simulink model "X8"  (R2020b)
settings: Solver=FixedStepAuto  StartTime=0.0  StopTime=Inf  FixedStep=1e-3  MinStep=0.0001  RelTol=1e-3  EnableMultiTasking=on
model workspace (MAT data in the model file):
  FaultMode = Simulink.Parameter
  FaultMode.Value = 0
  FaultMode.Description = 'Fault mode parameter object'
  FaultMode.DataType = 'auto'
  FaultMode.Dimensions = [1 1]
values from neighbouring files (symbols this model uses):
  A = [ ... (first row only)    [calc_sys_long.m]
  C_L_delta_eInterpolation = Create_interpolation(C_L_delta_e_data,'C_L_delta_e_data')    [coeff_ctrl.m]
  F = K * (-(C_D_0 + C_D_alpha * alpha) * cos(alpha)      + (C_L_O + C_L_alpha * alpha)*sin(alpha)) - f_x    [calc_alpha.m]
  h0 = 1000    [init.m]
  input_source = 4    [runX8.m]
  input_source0 = 1    [runX8.m]
  input_step_time = 0    [runX8.m]
  J = @(v_a, omega) 2 * pi * v_a / (omega*obj.prop_diam)    [kalmanFilters.m]    (also in motor.m = 2*pi*Va/omega/prop_diam; motor_fault.m = c2 / omega)
  lat0 = 37.6205    [init.m]
  lon0 = -122.3815    [init.m]
  P = filter.P(i,i,k_0:k_1)    [filterTest.m]    (also in kalmanFilters.m = filter.P)
  p = rate(1) + wind(4)    [forces.m]    (also in forces_trim.m)
  q = rate(2) + wind(5)    [forces.m]    (also in forces_trim.m)
  r = rate(3) + wind(6)    [forces.m]    (also in forces_trim.m)
  T_elevon2ailelev = [1 1 ... (first row only)    [init.m]
  Ts = 0.01    [init.m]
  U_trim = [op.Inputs(1).u;op.Inputs(2).u;op.Inputs(3).u;op.Inputs(4).u]    [X8Trim.m]
  x0 = X_trim    [X8Trim.m]    (also in init.m = [eta_0', ny_0' zeros(1,6)]'; runX8.m = [      0                 0                    -h_ini        ; trimX8.m = [      37.5                 0                    -h_ini     )
undefined symbols (not defined in the file or in its folder): Friction, ia, ib, interp_C_D_alpha, interp_C_D_delta_e, interp_C_D_q, interp_C_L_alpha, interp_C_l_beta, interp_C_l_delta_a, interp_C_L_delta_e, interp_C_l_delta_r, interp_C_l_p, interp_C_L_q, interp_C_l_r, interp_C_m_alpha, interp_C_m_delta_e, interp_C_m_q, interp_C_n_beta, interp_C_n_delta_a, interp_C_n_p, interp_C_n_r, interp_C_Y_beta, interp_C_Y_delta_a, interp_C_Y_delta_r, interp_C_Y_p, interp_C_Y_r, Ion, JSBSim, Light, Lithium, Lls, MIL, Prop_param, Rascal110, Receive, Rs, Send, Standard_Devices, thetam, UDP_Protocol, wm, x0_stationary
libraries: simulink_extras x15, simulink x8, aerolibwind2 x4, sldrtlib x3, aerolibfltsims x3, aerolibactuator x3, sharedtransform x3, electricdrivelib x2, dspnetwork x1, aerolibnav x1, sharedutil x1, powerlib_meascontrol x1
(part 1 of 2)
settings Model: SimulationMode=accelerator  PacingRate=10  ParameterArgumentNames=FaultMode  OrderedModelArguments=off  Creator=krisgry  LastModifiedBy=ole
settings SolverCC: ZeroCrossAlgorithm=Adaptive  AutoInsertRateTranBlk=on
settings DataIOCC: SaveOutput=off  DSMLogging=off  SaveTime=off  ReturnWorkspaceOutputs=off  LoggingFileName=simulationData.mat
settings OptimizationCC: EfficientMapNaN2IntZero=off  AccelVerboseBuild=on
settings DebuggingCC: ReadBeforeWriteMsg=DisableAll  WriteAfterWriteMsg=DisableAll  WriteAfterReadMsg=DisableAll  SolverPrmCheckMsg=warning  MultiTaskCondExecSysMsg=warning  SFUnexpectedBacktrackingDiag=warning  SFNoUnconditionalDefaultTransitionDiag=warning  SFExecutionAtInitializationDiag=none  ArithmeticOperatorsInVariantConditions=warning
settings HardwareCC: ProdBitPerLong=64  ProdHWDeviceType=Intel->x86-64 (Mac OS X)  TargetBitPerLong=64  TargetBitPerPointer=64  TargetBitPerSizeT=64  TargetBitPerPtrDiffT=64  TargetLongLongMode=on  TargetIntDivRoundTo=Zero  TargetEndianess=LittleEndian  TargetWordSize=64  TargetHWDeviceType=MATLAB Host  ProdEqTarget=off
settings ModelReferenceCC: PropagateSignalLabelsOutOfModel=off
settings SFSimCC: SimUseLocalCustomCode=off  CustomCodeUndefinedFunction=UseInterfaceOnly
settings CodeAppCC: MaxIdLength=128
settings GRTTargetCC: TargetLangStandard=C89/C90 (ANSI)  CombineOutputUpdateFcns=off  GRTInterface=on
settings ConfigComp: CovMetricSettings=dw  CovSaveCumulativeToWorkspaceVar=on  CovSaveSingleToWorkspaceVar=on  CovExternalEMLEnable=off  CovSFcnEnable=off

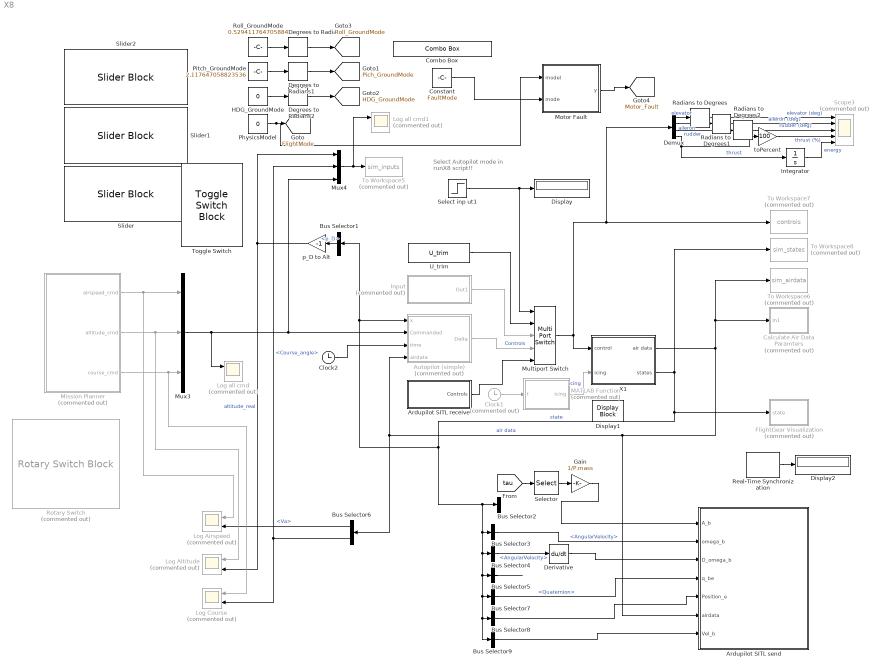
== system X8 ==
  note: Select Autopilot
      | mode in runX8 script!!
  Ardupilot SITL receive : Subsystem
  Ardupilot SITL send : Subsystem
  Autopilot (simple) : Subsystem  Commented=on
  Bus Selector1 : BusSelector  OutputSignals=Position.p_D
  Bus Selector2 : BusSelector  OutputSignals=Acceleration
  Bus Selector3 : BusSelector  OutputSignals=AngularVelocity
  Bus Selector4 : BusSelector  OutputSignals=AngularVelocity
  Bus Selector5 : BusSelector  OutputSignals=Velocity.u,Velocity.v,Velocity.w  OutputAsBus=on
  Bus Selector6 : BusSelector  OutputSignals=Va,Course_angle
  Bus Selector7 : BusSelector  OutputSignals=Quaternion
  Bus Selector8 : BusSelector  OutputSignals=Position.p_N,Position.p_E,Position.p_D  OutputAsBus=on
  Bus Selector9 : BusSelector  OutputSignals=Velocity.u,Velocity.v,Velocity.w  OutputAsBus=on
  Calculate Air Data Paramters : Subsystem  Commented=on
  Clock1 : Clock  Commented=on
  Clock2 : Clock
  Combo Box : ComboBox  LabelPosition=Hide  SelectedLabel=Mode 0
      settings: Values={{'Mode 0', 'Mode 1', 'Mode 2', 'Mode 3'}, [0 1 2 3]}
  Constant : Constant  Value=FaultMode
  Degrees to Radians : simulink_extras/Transformations/Degrees to Radians
  Degrees to Radians1 : simulink_extras/Transformations/Degrees to Radians
  Degrees to Radians2 : simulink_extras/Transformations/Degrees to Radians
  Demux : Demux
  Derivative : Derivative
  Display : Display
  Display1 : DisplayBlock
  Display2 : Display
  "FlightGear Visualization " : Subsystem  Commented=on
  Gain : Gain  Gain=1/P.mass
  HDG_GroundMode : Constant  Value=0  SampleTime=-1
  Input : Subsystem  Commented=on
  Integrator : Integrator
  Log Airspeed : Scope  Commented=on  NumInputPorts=2
  Log Altitude : Scope  Commented=on  NumInputPorts=2
  Log Course : Scope  Commented=on  NumInputPorts=2
  Log all cmd : Scope  Commented=on  NumInputPorts=2
  Log all cmd1 : Scope  Commented=on  NumInputPorts=2
  MATLAB Function : MATLAB Function  Commented=on  TreatAsAtomicUnit=on
  Mission Planner : Subsystem  Commented=on
  Motor Fault : MATLAB Function  TreatAsAtomicUnit=on
  Multiport Switch : MultiPortSwitch  Inputs=4
  Mux3 : Mux  Inputs=3
  Mux4 : Mux  Inputs=3
  PhysicsModel : Constant  Value=0  SampleTime=[0,1]
  Pitch_GroundMode : Constant  Value=2.117647058823536  SampleTime=-1
  Radians to Degrees : simulink_extras/Transformations/Radians to Degrees
  Radians to Degrees1 : simulink_extras/Transformations/Radians to Degrees
  Radians to Degrees2 : simulink_extras/Transformations/Radians to Degrees
  Real-Time Synchronization : sldrtlib/Real-Time Synchronization  SampleTime=0.1  MaxMissedTicks=inf  ShowMissedTicks=on  YieldWhenWaiting=off
  Roll_GroundMode : Constant  Value=0.529411764705884  SampleTime=-1
  Rotary Switch : RotarySwitchBlock  Commented=on
      settings: Values={{'Off', 'K_E', 'R_E', 'icing', 'off', 'I_0', 'c_v'}, [0 1 2 3 4 5 6]}
  Scope3 : Scope  Commented=on  NumInputPorts=5
  Select inp ut1 : Step  Time=input_step_time  Before=input_source0  After=input_source  SampleTime=0
  Selector : Selector  InputPortWidth=6  IndexOptions=Index vector (dialog)  Indices=[1 2 3]  OutputSizes=1
  Slider : SliderBlock  ScaleMax=360
  Slider1 : SliderBlock  ScaleMin=-180  ScaleMax=180
  Slider2 : SliderBlock  ScaleMin=-90  ScaleMax=90
  To Workspace5 : ToWorkspace  Commented=on  VariableName=sim_inputs  SaveFormat=Timeseries  SampleTime=-1
  To Workspace6 : ToWorkspace  Commented=on  VariableName=sim_airdata  SaveFormat=Timeseries  SampleTime=-1
  To Workspace7 : ToWorkspace  Commented=on  VariableName=controls  SaveFormat=Timeseries  SampleTime=-1
  To Workspace8 : ToWorkspace  Commented=on  VariableName=sim_states  SaveFormat=Timeseries  SampleTime=-1
  Toggle Switch : ToggleSwitchBlock
      settings: Values={{'Ground', 'Fly'}, [0 1]}
  U_trim : Constant  Value=U_trim  SampleTime=-1
  X1 : Subsystem
  p_D to Alt : Gain  Gain=-1
  toPercent : Gain  Gain=100
  tag scope: FlightMode=global, HDG_GroundMode=global, Motor_Fault=global, Pich_GroundMode=global, Roll_GroundMode=global
  wires:
  X1/1(air data) -> Autopilot (simple)/4(airdata), Bus Selector6/1, Ardupilot SITL send/6(airdata), Calculate Air Data Paramters/1(In1), To Workspace6/1  "air data"
  Multiport Switch/1 -> X1/1(control), To Workspace7/1, Demux/1
  U_trim/1 -> Multiport Switch/2
  Input/1(Out1) -> Multiport Switch/3
  X1/2(states) -> Bus Selector2/1, Bus Selector9/1, Bus Selector8/1, Bus Selector7/1, Bus Selector5/1, Bus Selector4/1, Bus Selector3/1, Bus Selector1/1, Autopilot (simple)/1(x), "FlightGear Visualization "/1(state), To Workspace8/1  "state"
  Select inp ut1/1 -> Multiport Switch/1, Display/1
  Mux3/1 -> Log all cmd/1, Mux4/3, Autopilot (simple)/2(Commanded)
  Autopilot (simple)/1(Delta) -> Multiport Switch/4  "Controls"
  Bus Selector6/2 -> Log Course/2, Mux4/2  "<Course_angle>"
  Bus Selector1/1 -> p_D to Alt/1  "<p_D>"
  p_D to Alt/1 -> Log Altitude/2, Mux4/1  "altitude_real"
  Mux4/1 -> Log all cmd1/1, To Workspace5/1
  Bus Selector6/1 -> Log Airspeed/2  "<Va>"
  Mission Planner/1(airspeed_cmd) -> Mux3/1, Log Airspeed/1
  Mission Planner/3(course_cmd) -> Log Course/1, Mux3/3
  Mission Planner/2(altitude_cmd) -> Log Altitude/1, Mux3/2
  Demux/1 -> Radians to Degrees/1  "elevator"
  Demux/2 -> Radians to Degrees1/1  "aileron"
  Demux/3 -> Radians to Degrees2/1  "rudder"
  Demux/4 -> Integrator/1, toPercent/1  "thrust"
  Integrator/1 -> Scope3/5  "energy"
  Bus Selector3/1 -> Ardupilot SITL send/2(omega_b)  "<AngularVelocity>"
  Bus Selector4/1 -> Derivative/1  "<AngularVelocity>"
  Bus Selector7/1 -> Ardupilot SITL send/4("q_be ")  "<Quaternion>"
  Bus Selector8/1 -> Ardupilot SITL send/5(Position_e)
  Derivative/1 -> Ardupilot SITL send/3(D_omega_b)
  Ardupilot SITL receive/1(Controls) -> Multiport Switch/5
  MATLAB Function/1(icing) -> X1/2(icing)  "icing"
  Clock1/1 -> MATLAB Function/1(t)
  Radians to Degrees/1 -> Scope3/1  "elevator (deg)"
  Radians to Degrees1/1 -> Scope3/2  "aileron (deg)"
  Radians to Degrees2/1 -> Scope3/3  "rudder (deg)"
  toPercent/1 -> Scope3/4  "thrust (%)"
  PhysicsModel/1 -> Motor Fault/1(model), [FlightMode]
  Pitch_GroundMode/1 -> Degrees to Radians1/1
  HDG_GroundMode/1 -> Degrees to Radians2/1
  Roll_GroundMode/1 -> Degrees to Radians/1
  Degrees to Radians/1 -> [Roll_GroundMode]
  Degrees to Radians1/1 -> [Pich_GroundMode]
  Degrees to Radians2/1 -> [HDG_GroundMode]
  Clock2/1 -> Autopilot (simple)/3(time)
  Gain/1 -> Ardupilot SITL send/1(A_b)
  Real-Time Synchronization/1 -> Display2/1
  Bus Selector5/1 -> ?
  Bus Selector9/1 -> Ardupilot SITL send/7(Vel_b)
  [tau] -> Selector/1
  Selector/1 -> Gain/1
  Motor Fault/1(y) -> [Motor_Fault]
  Constant/1 -> Motor Fault/2(mode)

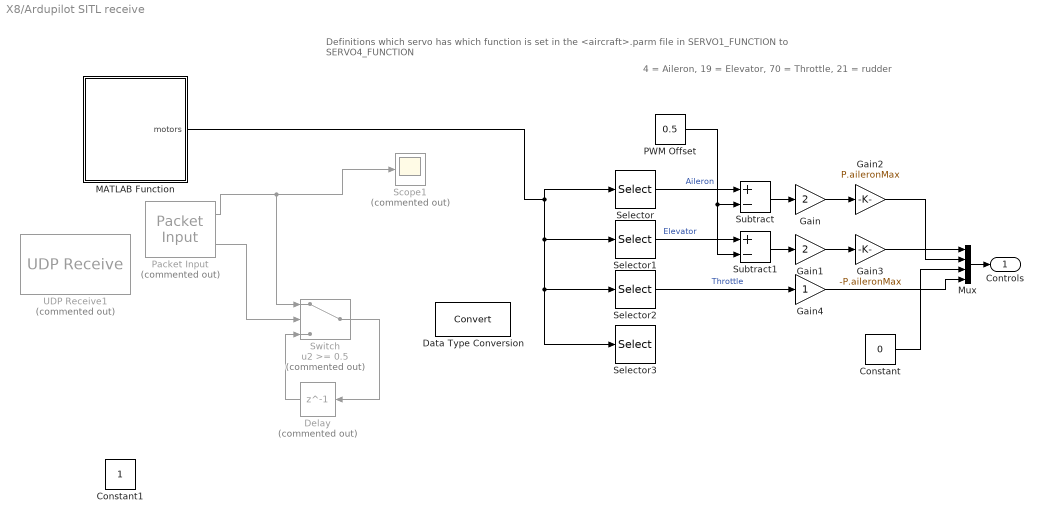
== system X8/Ardupilot SITL receive ==
  note: Definitions which servo has which function is set in the <aircraft>.parm file in SERVO1_FUNCTION to SERVO4_FUNCTION
  note: 4 = Aileron, 19 = Elevator, 70 = Throttle, 21 = rudder
  Constant : Constant  Value=0
  Constant1 : Constant
  Data Type Conversion : DataTypeConversion
  Delay : Delay  Commented=on  DelayLength=1  InitialCondition=0
  Gain : Gain  Gain=2
  Gain1 : Gain  Gain=2
  Gain2 : Gain  Gain=P.aileronMax
  Gain3 : Gain  Gain=-P.aileronMax
  Gain4 : Gain
  MATLAB Function : MATLAB Function  TreatAsAtomicUnit=on  SystemSampleTime=0.02
  Mux : Mux
  PWM Offset : Constant  Value=0.5
  Packet Input : sldrtlib/Packet Input  Commented=on  SampleTime=0.002  MaxMissedTicks=inf  ShowMissedTicks=off  YieldWhenWaiting=on  DrvName=Standard_Devices/UDP_Protocol  DrvAddress=9002  DrvOptions=[0 16385 0 0 0 0 0 0 0 0 0 0 0 0 0 0 0 0 0 0 0 0 0 0 0 0 0 0 0 0 0 0 0 0 0 0 0 0 0 0 0 0 0 0 0 0 0 0 0 0 0 0 0 0 0 0 0 0 0 0 0 0 0 0 0 0 0 0 0 0 0 0 0 0 0 0 0 0 0 0 0 0 0 0 0 0 0 0 0 0 0 0 0 0 0 0 0 0 0 0 0 0 0 0 0 0 0 0 0 0 0 0 0 0 0 0 0 0 0 0 0 0 0 0 0 0 0 0 0 0 0 0 0 0 0 0 0 0 0 0 0 0 0 0 0 0 0 0 0 0 0 0 0 0 0 0 0 0 0 0 0 0 0 0 0 0 0 0 0 0 0 0 0 0 0 0 0 0 0 0 0 0 0 0 0 0 0 0 0 0 0 0 0 0 0 0 0 0 0 0 0 0 0 0 0 0 0 0 0 0 0 0 0 0 0 0 0 0 0 0 0 0 0 0 0 0 0 0 0 0 0 0 0 0 0 0 0 0 0 0 0 0 0 0 0 0 0 0 0 0 0 0 0 0 0 0]  PacketSize=64  DataTypes='16*single'  ShowReady=on  ShowError=off  PacketID=1  ByteOrder=1  ShowTimestamp=off
      settings: AttributesFormatString=UDP Protocol [9002]
  Scope1 : Scope  Commented=on
  Selector : Selector  InputPortWidth=16  IndexOptions=Index vector (dialog)  Indices=1  OutputSizes=1
  Selector1 : Selector  InputPortWidth=16  IndexOptions=Index vector (dialog)  Indices=2  OutputSizes=1
  Selector2 : Selector  InputPortWidth=16  IndexOptions=Index vector (dialog)  Indices=3  OutputSizes=1
  Selector3 : Selector  InputPortWidth=16  IndexOptions=Index vector (dialog)  Indices=4  OutputSizes=1
  Subtract : Sum  Inputs=+-
  Subtract1 : Sum  Inputs=+-
  Switch : Switch  Commented=on  Threshold=0.5
  UDP Receive1 : dspnetwork/UDP Receive  Commented=on  localURL='0.0.0.0'  localPort=9002  remoteURL='127.0.0.1'  remotePort=-1  recvBufferSize=256  dims=16  signalDatatype=single  isComplex=off  isVarSize=off  showBlockingTime=on  blockingTime=0.02  sampletime=0.01  blockPlatform=HOST
  Controls : Outport  VectorParamsAs1DForOutWhenUnconnected=off
  wires:
  Selector2/1 -> Gain4/1  "Throttle"
  Mux/1 -> Controls/1
  Selector/1 -> Subtract/1  "Aileron"
  Selector1/1 -> Subtract1/1  "Elevator"
  PWM Offset/1 -> Subtract1/2, Subtract/2
  Subtract/1 -> Gain/1
  Subtract1/1 -> Gain1/1
  Gain1/1 -> Gain3/1
  Gain/1 -> Gain2/1
  Gain3/1 -> Mux/1
  Constant/1 -> Mux/3
  Gain2/1 -> Mux/2
  Gain4/1 -> Mux/4
  MATLAB Function/1(motors) -> Selector/1, Selector2/1, Selector3/1, Selector1/1
  Packet Input/1 -> Switch/1, Scope1/1
  Switch/1 -> Delay/1
  Packet Input/2 -> Switch/2
  Delay/1 -> Switch/3

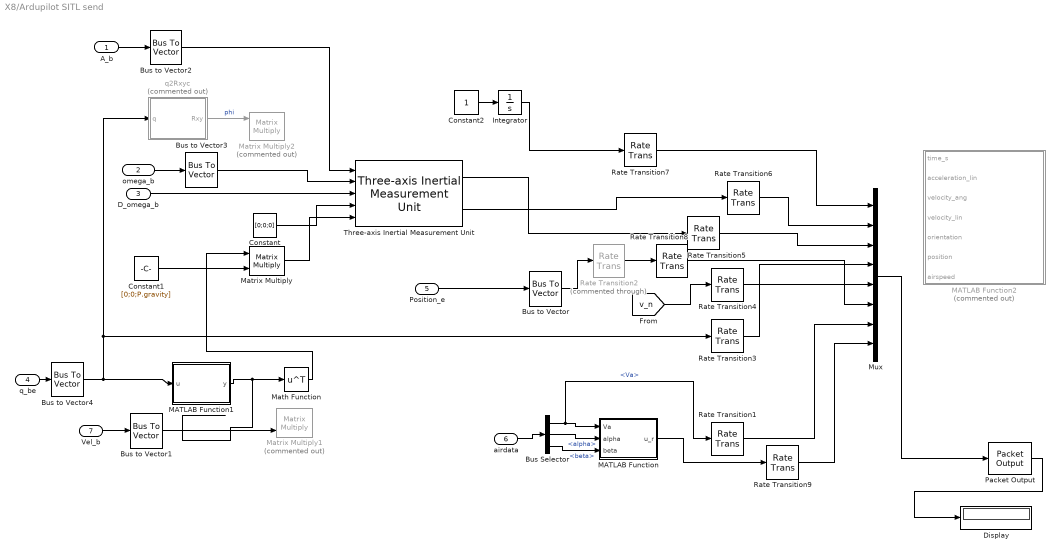
== system X8/Ardupilot SITL send ==
  A_b : Inport
  omega_b : Inport  Port=2
  D_omega_b : Inport  Port=3
  "q_be " : Inport  Port=4
  Position_e : Inport  Port=5
  airdata : Inport  Port=6
  Vel_b : Inport  Port=7
  Bus Selector : BusSelector  OutputSignals=Va,alpha,beta
  Bus to Vector{,1..4} (5 alike) : BusToVector
  Constant : Constant  Value=[0;0;0]
  Constant1 : Constant  Value=[0;0;P.gravity]
  Constant2 : Constant
  Display : Display
  Integrator : Integrator
  MATLAB Function : MATLAB Function  TreatAsAtomicUnit=on
  MATLAB Function1 : MATLAB Function  TreatAsAtomicUnit=on
  MATLAB Function2 : MATLAB Function  Commented=on  TreatAsAtomicUnit=on  SystemSampleTime=0.002
  Math Function : Math  Operator=transpose  SignedPower=on  SaturateOnIntegerOverflow=on
  Matrix Multiply : Product  Multiplication=Matrix(*)
  Matrix Multiply1 : Product  Commented=on  Multiplication=Matrix(*)
  Matrix Multiply2 : Product  Commented=on  Multiplication=Matrix(*)
  Mux : Mux  Inputs=8
  Packet Output : sldrtlib/Packet Output  SampleTime=0.002  MaxMissedTicks=inf  ShowMissedTicks=on  YieldWhenWaiting=off  DrvName=Standard_Devices/UDP_Protocol  DrvAddress=16384  DrvOptions=[0 9003 49 50 55 46 48 46 48 46 49 0 0 0 0 0 0 0 0 0 0 0 0 0 0 0 0 0 0 0 0 0 0 0 0 0 0 0 0 0 0 0 0 0 0 0 0 0 0 0 0 0 0 0 0 0 0 0 0 0 0 0 0 0 0 0 0 0 0 0 0 0 0 0 0 0 0 0 0 0 0 0 0 0 0 0 0 0 0 0 0 0 0 0 0 0 0 0 0 0 0 0 0 0 0 0 0 0 0 0 0 0 0 0 0 0 0 0 0 0 0 0 0 0 0 0 0 0 0 0 0 0 0 0 0 0 0 0 0 0 0 0 0 0 0 0 0 0 0 0 0 0 0 0 0 0 0 0 0 0 0 0 0 0 0 0 0 0 0 0 0 0 0 0 0 0 0 0 0 0 0 0 0 0 0 0 0 0 0 0 0 0 0 0 0 0 0 0 0 0 0 0 0 0 0 0 0 0 0 0 0 0 0 0 0 0 0 0 0 0 0 0 0 0 0 0 0 0 0 0 0 0 0 0 0 0 0 0 0 0 0 0 0 0 0 0 0 0 0 0 0 0 0 0 0 0]  PacketSize=176  DataTypes='22*double'  ShowReady=off  ShowError=off  PacketID=1  ByteOrder=1  InitialValue=[]  FinalValue=[]
      settings: AttributesFormatString=UDP Protocol [16384]
  Rate Transition{1,5..7} (4 alike) : RateTransition
  Rate Transition2 : RateTransition  Commented=through
  Rate Transition{3..4,8..9} (4 alike) : RateTransition  OutPortSampleTimeOpt=Inherit
  Three-axis Inertial Measurement Unit : aerolibnav/Three-axis Inertial Measurement Unit  units=Metric (MKS)  imu=[0 0 0]  i_Ts=0.001  dtype_a=off  w_a=190  z_a=0.707  a_sf_cc=[1 0 0; 0 1 0; 0 0 1]  a_bias=[0 0 0]  a_sat="[-inf  -inf  -inf  inf inf inf]"  dtype_g=off  w_g=190  z_g=0.707  g_sf_cc=[1 0 0; 0 1 0; 0 0 1]  g_bias=[0 0 0]  g_sens=[0 0 0]  g_sat="[-inf  -inf  -inf  inf inf inf]"  i_rand=off  i_seeds=[23093 23094 23095 23096 23097 23098]  i_pow=[0.001 0.001 0.001 0.0001 0.0001 0.0001]
  q2Rxyc : MATLAB Function  Commented=on  TreatAsAtomicUnit=on
  wires:
  Position_e/1 -> Bus to Vector/1
  airdata/1 -> Bus Selector/1
  Rate Transition2/1 -> Rate Transition8/1
  Bus Selector/1 -> Rate Transition1/1, MATLAB Function/1(Va)  "<Va>"
  A_b/1 -> Bus to Vector2/1
  D_omega_b/1 -> Three-axis Inertial Measurement Unit/3
  Constant/1 -> Three-axis Inertial Measurement Unit/4
  MATLAB Function1/1(y) -> Math Function/1
  Integrator/1 -> Rate Transition7/1
  Three-axis Inertial Measurement Unit/2 -> Rate Transition6/1
  Bus to Vector2/1 -> Three-axis Inertial Measurement Unit/1
  Constant1/1 -> Matrix Multiply/2
  Matrix Multiply/1 -> Three-axis Inertial Measurement Unit/5
  Bus to Vector/1 -> Rate Transition2/1
  Three-axis Inertial Measurement Unit/1 -> Rate Transition5/1
  Rate Transition7/1 -> Mux/1
  Rate Transition6/1 -> Mux/2
  Rate Transition5/1 -> Mux/3
  Rate Transition1/1 -> Mux/7
  Mux/1 -> Packet Output/1
  Packet Output/1 -> Display/1
  Bus Selector/2 -> MATLAB Function/2(alpha)  "<alpha>"
  Bus Selector/3 -> MATLAB Function/3(beta)  "<beta>"
  MATLAB Function/1(u_r) -> Rate Transition9/1
  Vel_b/1 -> Bus to Vector1/1
  ? -> Matrix Multiply1/1
  Bus to Vector1/1 -> Matrix Multiply1/2
  [v_n] -> Rate Transition4/1
  Constant2/1 -> Integrator/1
  Math Function/1 -> Matrix Multiply/1
  q2Rxyc/1(Rxy) -> Matrix Multiply2/1  "phi"
  omega_b/1 -> Bus to Vector3/1
  Bus to Vector3/1 -> Three-axis Inertial Measurement Unit/2
  "q_be "/1 -> Bus to Vector4/1
  Bus to Vector4/1 -> MATLAB Function1/1(u), q2Rxyc/1(q), Rate Transition3/1
  Rate Transition3/1 -> Mux/4
  Rate Transition8/1 -> Mux/6
  Rate Transition4/1 -> Mux/5
  Rate Transition9/1 -> Mux/8

== system X8/Autopilot (simple) ==
  x : Inport
  Commanded : Inport  Port=2
  time : Inport  Port=3
  airdata : Inport  Port=4
  Bus Selector : BusSelector  OutputSignals=Va,alpha,beta,wind_x,wind_y,wind_z,Course_angle
  Bus Selector1 : BusSelector  OutputSignals=Position.p_N,Position.p_E,Position.p_D,Velocity.u,Velocity.v,Velocity.w,Attitude.phi,Attitude.theta,Attitude.psi,AngularVelocity.p,AngularVelocity.q,AngularVelocity.r
  Delay : Delay  DelayLength=1  InitialCondition="[x0(1:3);  x0(8:10); zeros(3,1); x0(11:13); zeros(11,1)]"  SampleTime=Ts
  Interpreted MATLAB Function : MATLABFcn  MATLABFcn=autopilot  OutputDimensions=4
  Memory : Memory  Commented=on  InitialCondition="[x0(1:3);  x0(8:10); zeros(3,1); x0(11:13); zeros(11,1)]"
  Mux : Mux
  Mux1 : Mux  Inputs=7
  Mux2 : Mux  Inputs=12
  To Workspace1 : ToWorkspace  VariableName=commanded  SaveFormat=Structure With Time  SampleTime=-1
  To Workspace2 : ToWorkspace  VariableName=delta  SaveFormat=Structure With Time  SampleTime=-1
  Delta : Outport  VectorParamsAs1DForOutWhenUnconnected=off
  wires:
  Commanded/1 -> To Workspace1/1, Mux/2
  Mux/1 -> Delay/1
  time/1 -> Mux/4
  airdata/1 -> Bus Selector/1
  Bus Selector/1 -> Mux1/1  "<Va>"
  Bus Selector/2 -> Mux1/2  "<alpha>"
  Bus Selector/3 -> Mux1/3  "<beta>"
  Bus Selector/4 -> Mux1/4  "<wind_x>"
  Bus Selector/5 -> Mux1/5  "<wind_y>"
  Bus Selector/6 -> Mux1/6  "<wind_z>"
  Mux1/1 -> Mux/3
  x/1 -> Bus Selector1/1
  Bus Selector1/1 -> Mux2/1  "<p_N>"
  Bus Selector1/2 -> Mux2/2  "<p_E>"
  Bus Selector1/4 -> Mux2/4  "<u>"
  Bus Selector1/3 -> Mux2/3  "<p_D>"
  Bus Selector1/5 -> Mux2/5  "<v>"
  Bus Selector1/6 -> Mux2/6  "<w>"
  Bus Selector1/7 -> Mux2/7  "<phi>"
  Bus Selector1/9 -> Mux2/9  "<psi>"
  Bus Selector1/8 -> Mux2/8  "<theta>"
  Bus Selector1/10 -> Mux2/10  "<p>"
  Bus Selector1/11 -> Mux2/11  "<q>"
  Bus Selector1/12 -> Mux2/12  "<r>"
  Mux2/1 -> Mux/1
  Interpreted MATLAB Function/1 -> To Workspace2/1, Delta/1
  Delay/1 -> Interpreted MATLAB Function/1
  Bus Selector/7 -> Mux1/7  "<Course_angle>"

== system X8/Calculate Air Data Paramters ==
  In1 : Inport
  Bus Selector : BusSelector  OutputSignals=alpha,beta,Va
  Radians to Degrees1 : simulink_extras/Transformations/Radians to Degrees
  Radians to Degrees4 : simulink_extras/Transformations/Radians to Degrees
  To Workspace : ToWorkspace  VariableName=alpha  SaveFormat=Structure With Time  SampleTime=-1
  To Workspace1 : ToWorkspace  VariableName=beta  SaveFormat=Structure With Time  SampleTime=-1
  To Workspace2 : ToWorkspace  VariableName=va  SaveFormat=Structure With Time  SampleTime=-1
  wires:
  Radians to Degrees1/1 -> To Workspace1/1  "beta_ref"
  Radians to Degrees4/1 -> To Workspace/1  "alpha_ref"
  In1/1 -> Bus Selector/1
  Bus Selector/2 -> Radians to Degrees1/1  "<beta>"
  Bus Selector/1 -> Radians to Degrees4/1  "<alpha>"
  Bus Selector/3 -> To Workspace2/1  "<Va>"

== system X8/FlightGear Visualization  ==
  state : Inport
  Bus Selector : BusSelector  OutputSignals=Attitude  OutputAsBus=on
  Bus Selector2 : BusSelector  OutputSignals=Position
  "FlatEarth to Lon/Lat/Alt " : Subsystem
  FlightGear Preconfigured 6DoF Animation : aerolibfltsims/FlightGear Preconfigured 6DoF Animation  xFlightGearVersion=v2018.1  DestinationIpAddress=127.0.0.1  DestinationPort=5600  SampleTime=0.02  packetVersion=24
  Generate Run Script : aerolibfltsims/Generate Run Script  Architecture=Linux  dataFlow=Send  GeometryModelName=Rascal110-JSBSim  AirportId=KSFO  RunwayId=10L  InitialAltitude=7224  InitialHeading=113  OffsetDistance=4.72  OffsetAzimuth=0  InstallScenery=off  DisableShaders=off  OriginAddress=127.0.0.1  DestinationPort=5600  OriginPort=5505  LocalAddress=127.0.0.1  OutputFileName=runfg.sh  FlightGearBaseDirectory=/home/adrian/.fgfs
  "Initial position (lon (°), lat (°), alt (m)) " : Constant  Value=[lon0, lat0, h0]  VectorParams1D=off
  Mux : Mux  Inputs=2
  wires:
  Mux/1 -> FlightGear Preconfigured 6DoF Animation/1
  Bus Selector2/1 -> "FlatEarth to Lon/Lat/Alt "/1("DeltaPosition [N (m), E(m), D(m)]")  "<Position>"
  state/1 -> Bus Selector2/1, Bus Selector/1
  "FlatEarth to Lon/Lat/Alt "/1(Out1) -> Mux/1
  Bus Selector/1 -> Mux/2  "<signal2>"
  "Initial position (lon (°), lat (°), alt (m)) "/1 -> "FlatEarth to Lon/Lat/Alt "/2("InitPosition [N (°), E(°), Alt (m)] ")

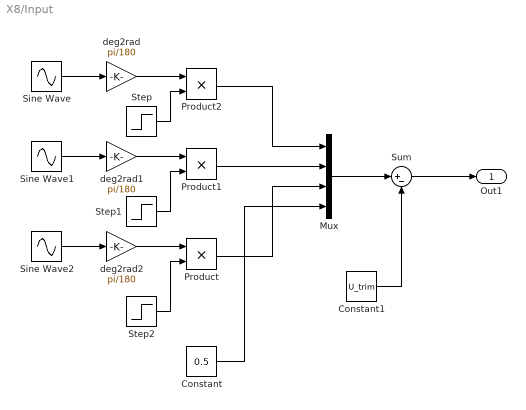
== system X8/Input ==
  Constant : Constant  Value=0.5
  Constant1 : Constant  Value=U_trim
  Mux : Mux
  Product : Product
  Product1 : Product
  Product2 : Product
  Sine Wave : Sin  Amplitude=1e-3  Frequency=0.1  SampleTime=0
  Sine Wave1 : Sin  Amplitude=1e-4  Frequency=0.01  Phase=pi/2  SampleTime=0
  Sine Wave2 : Sin  Amplitude=1e-3  Frequency=0.05  Phase=pi  SampleTime=0
  Step : Step  SampleTime=0
  Step1 : Step  Time=50  SampleTime=0
  Step2 : Step  Time=100  SampleTime=0
  Sum : Sum  Inputs=|+-
  deg2rad : Gain  Gain=pi/180
  deg2rad1 : Gain  Gain=pi/180
  deg2rad2 : Gain  Gain=pi/180
  Out1 : Outport  VectorParamsAs1DForOutWhenUnconnected=off
  wires:
  Sine Wave/1 -> deg2rad/1
  Sine Wave1/1 -> deg2rad1/1
  Sine Wave2/1 -> deg2rad2/1
  deg2rad2/1 -> Product/1
  deg2rad1/1 -> Product1/1
  deg2rad/1 -> Product2/1
  Step/1 -> Product2/2
  Step1/1 -> Product1/2
  Step2/1 -> Product/2
  Product2/1 -> Mux/1
  Product1/1 -> Mux/2
  Product/1 -> Mux/3
  Constant/1 -> Mux/4
  Mux/1 -> Sum/1
  Sum/1 -> Out1/1
  Constant1/1 -> Sum/2

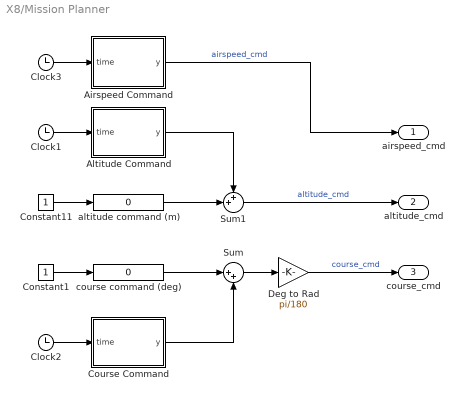
== system X8/Mission Planner ==
  "Airspeed Command " : MATLAB Function  TreatAsAtomicUnit=on
  Altitude Command : MATLAB Function  TreatAsAtomicUnit=on
  Clock1 : Clock
  Clock2 : Clock
  Clock3 : Clock
  Constant1 : Constant
  Constant11 : Constant
  "Course Command " : MATLAB Function  TreatAsAtomicUnit=on
  Deg to Rad : Gain  Gain=pi/180
  Sum : Sum  Inputs=|++
  Sum1 : Sum  Inputs=++|
  altitude command (m) : simulink/Math Operations/Slider Gain  gain=0  low=0  high=500
  course command (deg) : simulink/Math Operations/Slider Gain  gain=0  low=0  high=360
  airspeed_cmd : Outport  VectorParamsAs1DForOutWhenUnconnected=off
  altitude_cmd : Outport  Port=2  VectorParamsAs1DForOutWhenUnconnected=off
  course_cmd : Outport  Port=3  VectorParamsAs1DForOutWhenUnconnected=off
  wires:
  "Course Command "/1(y) -> Sum/2
  course command (deg)/1 -> Sum/1
  Sum1/1 -> altitude_cmd/1  "altitude_cmd"
  altitude command (m)/1 -> Sum1/2
  Sum/1 -> Deg to Rad/1
  Deg to Rad/1 -> course_cmd/1  "course_cmd"
  Constant11/1 -> altitude command (m)/1
  Constant1/1 -> course command (deg)/1
  "Airspeed Command "/1(y) -> airspeed_cmd/1  "airspeed_cmd"
  Clock3/1 -> "Airspeed Command "/1(time)
  Clock1/1 -> Altitude Command/1(time)
  Altitude Command/1(y) -> Sum1/1
  Clock2/1 -> "Course Command "/1(time)

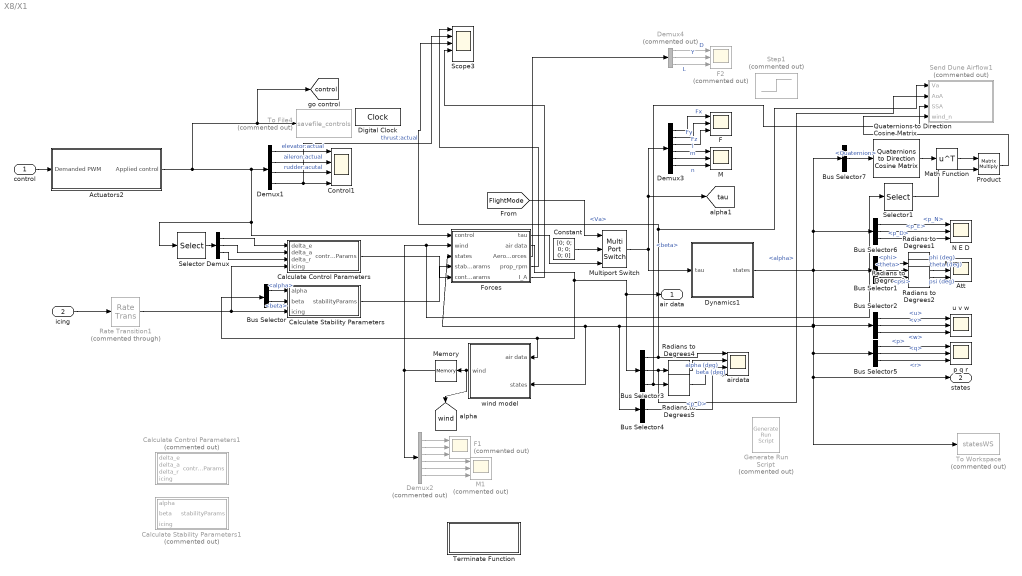
== system X8/X1 ==
  control : Inport
  icing : Inport  Port=2
  Actuators2 : Subsystem
  Att : Scope  NumInputPorts=3
  Bus Selector : BusSelector  OutputSignals=alpha,beta
  Bus Selector1 : BusSelector  OutputSignals=Attitude.phi,Attitude.theta,Attitude.psi
  Bus Selector2 : BusSelector  OutputSignals=Velocity.u,Velocity.v,Velocity.w
  Bus Selector3 : BusSelector  OutputSignals=Va,alpha,beta
  Bus Selector4 : BusSelector  OutputSignals=Position.p_D
  Bus Selector5 : BusSelector  OutputSignals=AngularVelocity.p,AngularVelocity.q,AngularVelocity.r
  Bus Selector6 : BusSelector  OutputSignals=Position.p_N,Position.p_E,Position.p_D
  Bus Selector7 : BusSelector  OutputSignals=Quaternion
  Calculate Control Parameters : Subsystem
  Calculate Control Parameters1 : Subsystem  Commented=on
  Calculate Stability Parameters : Subsystem
  Calculate Stability Parameters1 : Subsystem  Commented=on
  Constant : Constant  Value=[0; 0; 0; 0; 0; 0]
  Control1 : Scope  NumInputPorts=4
  Demux : Demux  Outputs=3
  Demux1 : Demux
  Demux2 : Demux  Commented=on  Outputs=6
  Demux3 : Demux  Outputs=6
  Demux4 : Demux  Commented=on  Outputs=3
  Digital Clock : DigitalClock  SampleTime=0.1
  Dynamics1 : Subsystem
  F : Scope  NumInputPorts=3
  F1 : Scope  Commented=on  NumInputPorts=3
  F2 : Scope  Commented=on  NumInputPorts=3
  Forces : Subsystem
  Generate Run Script : aerolibfltsims/Generate Run Script  Commented=on  Architecture=Win64  dataFlow=Send-Receive  GeometryModelName=x8  AirportId=KSFO  RunwayId=10L  InitialAltitude=7224  InitialHeading=113  OffsetDistance=4.72  OffsetAzimuth=0  InstallScenery=off  DisableShaders=off  OriginAddress=78.91.7.39  DestinationPort=5502  OriginPort=5505  LocalAddress=129.241.154.164  OutputFileName=runfg.sh  FlightGearBaseDirectory=/usr/share/flightgear
  M : Scope  NumInputPorts=3
  M1 : Scope  Commented=on  NumInputPorts=3
  Math Function : Math  Operator=transpose  SignedPower=on  SaturateOnIntegerOverflow=on
  Memory : Memory  InheritSampleTime=on
  Multiport Switch : MultiPortSwitch  DataPortOrder=Zero-based contiguous  Inputs=2  zeroidx=on
  N E D : Scope  NumInputPorts=3
  Product : Product  Multiplication=Matrix(*)
  Quaternions to Direction Cosine Matrix : sharedtransform/Quaternions to  Direction Cosine Matrix  aMode=aMode
      settings: SourceProductBaseCode=AE,PW,MT,UV,VE,VP
  Radians to Degrees{1..5} (5 alike) : simulink_extras/Transformations/Radians to Degrees
  Rate Transition1 : RateTransition  Commented=through  OutPortSampleTime=1
  Scope3 : Scope  NumInputPorts=5
  Selector : Selector  InputPortWidth=4  IndexOptions=Index vector (dialog)  Indices=[1 2 3]  OutputSizes=1
  Selector1 : Selector  InputPortWidth=6  IndexOptions=Index vector (dialog)  Indices=[1 2 3]  OutputSizes=1
  Send Dune Airflow1 : MATLAB Function  Commented=on  TreatAsAtomicUnit=on
  Step1 : Step  Commented=on  Time=0  Before=1  After=0  SampleTime=0
  Terminate Function : Subsystem  TreatAsAtomicUnit=on
  To File4 : ToFile  Commented=on  Filename=savefile_controls  MatrixName=sim_controls  SaveFormat=Timeseries  SampleTime=0.1
  To Workspace : ToWorkspace  Commented=on  VariableName=statesWS  SaveFormat=Timeseries  SampleTime=-1
  airdata : Scope  NumInputPorts=4
  p q r : Scope  NumInputPorts=3
  u v w : Scope  NumInputPorts=3
  wind model : Subsystem
  air data : Outport  VectorParamsAs1DForOutWhenUnconnected=off
  states : Outport  Port=2  VectorParamsAs1DForOutWhenUnconnected=off
  tag scope: control=global, tau=global, wind=global
  wires:
  Demux3/1 -> F/1  "Fx"
  Demux3/2 -> F/2  "Fy"
  Demux3/3 -> F/3  "Fz"
  Demux3/4 -> M/1  "l"
  Demux3/5 -> M/2  "m"
  Demux3/6 -> M/3  "n"
  Bus Selector2/1 -> u v w/1  "<u>"
  Bus Selector2/2 -> u v w/2  "<v>"
  Bus Selector2/3 -> u v w/3  "<w>"
  control/1 -> Actuators2/1(Demanded PWM)
  Bus Selector1/1 -> Radians to Degrees1/1  "<phi>"
  Bus Selector1/3 -> Radians to Degrees3/1  "<psi>"
  Bus Selector1/2 -> Radians to Degrees2/1  "<theta>"
  Radians to Degrees1/1 -> Att/1  "phi (deg)"
  Radians to Degrees2/1 -> Att/2  "theta (deg)"
  Radians to Degrees3/1 -> Att/3  "psi (deg)"
  Bus Selector3/1 -> Send Dune Airflow1/1(Va), Scope3/3, airdata/1  "<Va>"
  Bus Selector4/1 -> airdata/4  "<p_D>"
  Bus Selector3/2 -> Send Dune Airflow1/2(AoA), Radians to Degrees4/1  "<alpha>"
  Radians to Degrees4/1 -> airdata/2  "alpha (deg)"
  Demux1/4 -> Scope3/2, Control1/4  "thrust:actual"
  Demux1/2 -> Control1/2  "aileron:actual"
  Demux1/1 -> Control1/1  "elevator:actual"
  Demux2/1 -> F1/1
  Demux2/2 -> F1/2
  Demux2/3 -> F1/3
  Demux2/4 -> M1/1
  Demux2/5 -> M1/2
  Demux2/6 -> M1/3
  Bus Selector5/1 -> p q r/1  "<p>"
  Bus Selector5/2 -> p q r/2  "<q>"
  Bus Selector5/3 -> p q r/3  "<r>"
  Memory/1 -> Demux2/1, Selector1/1, Forces/2(wind)
  wind model/1(wind) -> [wind], Memory/1
  Bus Selector6/1 -> N E D/1  "<p_N>"
  Bus Selector6/2 -> N E D/2  "<p_E>"
  Bus Selector6/3 -> N E D/3  "<p_D>"
  Dynamics1/1(states) -> Bus Selector7/1, Bus Selector6/1, Bus Selector1/1, To Workspace/1, states/1, Bus Selector5/1, Bus Selector4/1, Forces/3(states), wind model/2(states), Bus Selector2/1
  Calculate Stability Parameters/1(stabilityParams) -> Forces/4(stabilityParams)
  icing/1 -> Rate Transition1/1
  Forces/3(AerodynamicForces) -> Demux4/1
  Demux4/2 -> F2/2  "Y"
  Demux4/1 -> F2/1  "D"
  Demux4/3 -> F2/3  "L"
  Demux1/3 -> Control1/3  "rudder:acutal"
  Bus Selector3/3 -> Radians to Degrees5/1, Send Dune Airflow1/3(SSA)  "<beta>"
  Radians to Degrees5/1 -> airdata/3  "beta (deg)"
  Multiport Switch/1 -> Dynamics1/1(tau), [tau], Demux3/1
  Constant/1 -> Multiport Switch/2
  [FlightMode] -> Multiport Switch/1
  Demux/1 -> Calculate Control Parameters/1("delta_e ")
  Demux/2 -> Calculate Control Parameters/2(delta_a)
  Demux/3 -> Calculate Control Parameters/3("delta_r ")
  Forces/1(tau) -> Multiport Switch/3
  Actuators2/1(Applied control) -> Demux1/1, Selector/1, Forces/1(control), To File4/1, [control]
  Rate Transition1/1 -> Calculate Control Parameters/4(icing), Calculate Stability Parameters/3(icing)
  Calculate Control Parameters/1(controlParams) -> Forces/5(controlParams)
  Forces/4(prop_rpm) -> Scope3/1
  Forces/5(I_A) -> Scope3/4
  Product/1 -> Send Dune Airflow1/4(wind_n)
  Forces/2(air data) -> air data/1, Bus Selector3/1, Bus Selector/1, wind model/1(air data)
  Bus Selector/2 -> Calculate Stability Parameters/2(beta)  "<beta>"
  Bus Selector/1 -> Calculate Stability Parameters/1("alpha ")  "<alpha>"
  Selector/1 -> Demux/1
  Bus Selector7/1 -> Quaternions to Direction Cosine Matrix/1  "<Quaternion>"
  Quaternions to Direction Cosine Matrix/1 -> Math Function/1
  Selector1/1 -> Product/2
  Math Function/1 -> Product/1

== system X8/FlightGear Visualization /FlatEarth to Lon//Lat//Alt  ==
  "DeltaPosition [N (m), E(m), D(m)]" : Inport
  "InitPosition [N (°), E(°), Alt (m)] " : Inport  Port=2
  Add : Sum  Inputs=2
  Demux : Demux  Outputs=3
  Divide : Product  Inputs=*/
  Divide1 : Product  Inputs=/*
  Earth Radius : Constant  Value=6378160
  Radians to Degrees : simulink_extras/Transformations/Radians to Degrees
  Radians to Degrees1 : simulink_extras/Transformations/Radians to Degrees
  Trigonometric Function : Trigonometry  Operator=asin
  Trigonometric Function1 : Trigonometry  Operator=asin
  Unary Minus : UnaryMinus
  Vector Concatenate : Concatenate  NumInputs=3
  Out1 : Outport  VectorParamsAs1DForOutWhenUnconnected=off
  wires:
  "DeltaPosition [N (m), E(m), D(m)]"/1 -> Demux/1
  Earth Radius/1 -> Divide1/1, Divide/2
  Divide/1 -> Trigonometric Function/1
  Demux/2 -> Divide1/2
  Divide1/1 -> Trigonometric Function1/1
  Demux/3 -> Unary Minus/1
  Unary Minus/1 -> Vector Concatenate/3
  "InitPosition [N (°), E(°), Alt (m)] "/1 -> Add/2
  Vector Concatenate/1 -> Add/1
  Add/1 -> Out1/1
  Demux/1 -> Divide/1
  Trigonometric Function/1 -> Radians to Degrees/1
  Trigonometric Function1/1 -> Radians to Degrees1/1
  Radians to Degrees1/1 -> Vector Concatenate/1
  Radians to Degrees/1 -> Vector Concatenate/2

== system X8/X1/Actuators2 ==
  Demanded PWM : Inport
  Actuator dynamics : Subsystem
  Demux : Demux  Outputs=[2,1,1]
  Demux1 : Demux
  Demux2 : Demux  Outputs=2
  Mux1 : Mux  Inputs=2
  Mux5 : Mux  Inputs=3
  PWM lookup : Subsystem  Commented=through
  Scale to [-1..1] : Subsystem
  Scale to [0..1] : Subsystem
  Scope1 : Scope  NumInputPorts=2
  Scope2 : Scope  NumInputPorts=3
  elevator-aileron to elevon : Gain  Gain=inv(T_elevon2ailelev)  Multiplication=Matrix(K*u) (u vector)
  elevon to elevator-aileron : Gain  Gain=T_elevon2ailelev  Multiplication=Matrix(K*u) (u vector)
  Applied control : Outport  PortDimensions=4  VectorParamsAs1DForOutWhenUnconnected=off
  wires:
  Mux5/1 -> Applied control/1, Demux1/1
  [prop_torque] -> Actuator dynamics/5(Prop torque)
  Actuator dynamics/4(Applied motor speed) -> Scale to [0..1]/1(prop speed)
  Demux1/1 -> Scope2/1
  Demux1/2 -> Scope2/2
  Demux1/4 -> Scope2/3
  Scale to [-1..1]/1(scaled deflection) -> elevon to elevator-aileron/1
  elevon to elevator-aileron/1 -> Mux5/1
  Actuator dynamics/3(Applied rudder) -> Mux5/2
  Scale to [0..1]/1(scaled prop speed) -> Mux5/3
  elevator-aileron to elevon/1 -> Demux2/1
  Actuator dynamics/1(Applied R elevon) -> Scope1/1, Mux1/1
  Mux1/1 -> Scale to [-1..1]/1(deflection)
  Actuator dynamics/2(Applied L elevon) -> Scope1/2, Mux1/2
  Demux/1 -> elevator-aileron to elevon/1
  PWM lookup/3(rud deflection) -> Actuator dynamics/3(Demanded rudder deflection1)
  PWM lookup/4(thrust) -> Actuator dynamics/4(Demanded motor speed)
  PWM lookup/2(Lservo deflection) -> Actuator dynamics/2("Demanded L elevon deflection ")
  PWM lookup/1(Rservo deflection) -> Actuator dynamics/1(Demanded R elevon deflection)
  Demux2/1 -> PWM lookup/1(Rservo PWM)
  Demux2/2 -> PWM lookup/2(Lservo)
  Demux/2 -> PWM lookup/3(Rudder)
  Demux/3 -> PWM lookup/4(thr pwm)
  Demanded PWM/1 -> Demux/1

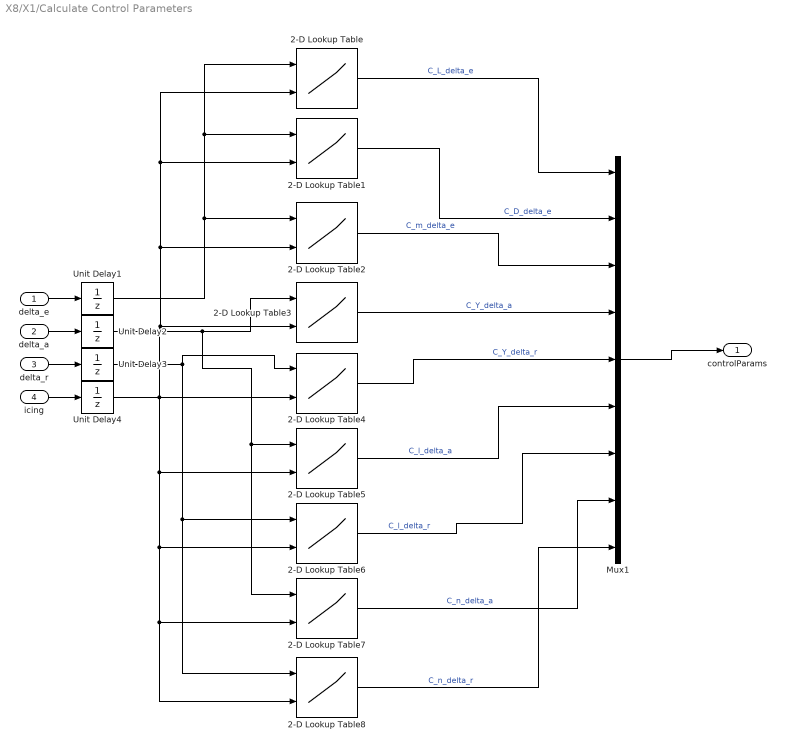
== system X8/X1/Calculate Control Parameters ==
  "delta_e " : Inport
  delta_a : Inport  Port=2
  "delta_r " : Inport  Port=3
  icing : Inport  Port=4
  2-D Lookup Table : Lookup_n-D  DataSpecification=Lookup table object  LookupTableObject=C_L_delta_eInterpolation  BreakpointsForDimension1=C_L_delta_eInterpolation.Points(:,1)  BreakpointsForDimension2=C_L_delta_eInterpolation.Points(:,2)  BreakpointsForDimension1FirstPoint=4  BreakpointsForDimension2FirstPoint=2  IndexSearchMethod=Linear search  Table=C_L_delta_eInterpolation.Values  ExtrapMethod=Clip  InternalRulePriority=Speed  RndMeth=Simplest  InputSameDT=on
      settings: InputPortMap=u0,u1
  2-D Lookup Table1 : Lookup_n-D  DataSpecification=Lookup table object  LookupTableObject=C_D_delta_eInterpolation  BreakpointsForDimension1=C_L_delta_eInterpolation.Points(:,1)  BreakpointsForDimension2=C_L_delta_eInterpolation.Points(:,2)  BreakpointsForDimension1FirstPoint=4  BreakpointsForDimension2FirstPoint=2  IndexSearchMethod=Linear search  Table=C_L_delta_eInterpolation.Values  ExtrapMethod=Clip  InternalRulePriority=Speed  RndMeth=Simplest  InputSameDT=on
      settings: InputPortMap=u0,u1
  2-D Lookup Table2 : Lookup_n-D  DataSpecification=Lookup table object  LookupTableObject=C_m_delta_eInterpolation  BreakpointsForDimension1=C_L_delta_eInterpolation.Points(:,1)  BreakpointsForDimension2=C_L_delta_eInterpolation.Points(:,2)  BreakpointsForDimension1FirstPoint=4  BreakpointsForDimension2FirstPoint=2  IndexSearchMethod=Linear search  Table=C_L_delta_eInterpolation.Values  ExtrapMethod=Clip  InternalRulePriority=Speed  RndMeth=Simplest  InputSameDT=on
      settings: InputPortMap=u0,u1
  2-D Lookup Table3 : Lookup_n-D  DataSpecification=Lookup table object  LookupTableObject=C_Y_delta_aInterpolation  BreakpointsForDimension1=C_L_delta_eInterpolation.Points(:,1)  BreakpointsForDimension2=C_L_delta_eInterpolation.Points(:,2)  BreakpointsForDimension1FirstPoint=4  BreakpointsForDimension2FirstPoint=2  IndexSearchMethod=Linear search  Table=C_L_delta_eInterpolation.Values  ExtrapMethod=Clip  InternalRulePriority=Speed  RndMeth=Simplest  InputSameDT=on
      settings: InputPortMap=u0,u1
  2-D Lookup Table4 : Lookup_n-D  DataSpecification=Lookup table object  LookupTableObject=C_Y_delta_rInterpolation  BreakpointsForDimension1=C_L_delta_eInterpolation.Points(:,1)  BreakpointsForDimension2=C_L_delta_eInterpolation.Points(:,2)  BreakpointsForDimension1FirstPoint=4  BreakpointsForDimension2FirstPoint=2  IndexSearchMethod=Linear search  Table=C_L_delta_eInterpolation.Values  ExtrapMethod=Clip  InternalRulePriority=Speed  RndMeth=Simplest  InputSameDT=on
      settings: InputPortMap=u0,u1
  2-D Lookup Table5 : Lookup_n-D  DataSpecification=Lookup table object  LookupTableObject=C_l_delta_aInterpolation  BreakpointsForDimension1=C_L_delta_eInterpolation.Points(:,1)  BreakpointsForDimension2=C_L_delta_eInterpolation.Points(:,2)  BreakpointsForDimension1FirstPoint=4  BreakpointsForDimension2FirstPoint=2  IndexSearchMethod=Linear search  Table=C_L_delta_eInterpolation.Values  ExtrapMethod=Clip  InternalRulePriority=Speed  RndMeth=Simplest  InputSameDT=on
      settings: InputPortMap=u0,u1
  2-D Lookup Table6 : Lookup_n-D  DataSpecification=Lookup table object  LookupTableObject=C_l_delta_rInterpolation  BreakpointsForDimension1=C_L_delta_eInterpolation.Points(:,1)  BreakpointsForDimension2=C_L_delta_eInterpolation.Points(:,2)  BreakpointsForDimension1FirstPoint=4  BreakpointsForDimension2FirstPoint=2  IndexSearchMethod=Linear search  Table=C_L_delta_eInterpolation.Values  ExtrapMethod=Clip  InternalRulePriority=Speed  RndMeth=Simplest  InputSameDT=on
      settings: InputPortMap=u0,u1
  2-D Lookup Table7 : Lookup_n-D  DataSpecification=Lookup table object  LookupTableObject=C_n_delta_aInterpolation  BreakpointsForDimension1=C_L_delta_eInterpolation.Points(:,1)  BreakpointsForDimension2=C_L_delta_eInterpolation.Points(:,2)  BreakpointsForDimension1FirstPoint=4  BreakpointsForDimension2FirstPoint=2  IndexSearchMethod=Linear search  Table=C_L_delta_eInterpolation.Values  ExtrapMethod=Clip  InternalRulePriority=Speed  RndMeth=Simplest  InputSameDT=on
      settings: InputPortMap=u0,u1
  2-D Lookup Table8 : Lookup_n-D  DataSpecification=Lookup table object  LookupTableObject=C_n_delta_rInterpolation  BreakpointsForDimension1=C_L_delta_eInterpolation.Points(:,1)  BreakpointsForDimension2=C_L_delta_eInterpolation.Points(:,2)  BreakpointsForDimension1FirstPoint=4  BreakpointsForDimension2FirstPoint=2  IndexSearchMethod=Linear search  Table=C_L_delta_eInterpolation.Values  ExtrapMethod=Clip  InternalRulePriority=Speed  RndMeth=Simplest  InputSameDT=on
      settings: InputPortMap=u0,u1
  Mux1 : Mux  Inputs=9
  Unit Delay{1..4} (4 alike) : UnitDelay  SampleTime=-1  HasFrameUpgradeWarning=on
  controlParams : Outport  VectorParamsAs1DForOutWhenUnconnected=off
  wires:
  Mux1/1 -> controlParams/1
  "delta_e "/1 -> Unit Delay1/1
  delta_a/1 -> Unit Delay2/1
  "delta_r "/1 -> Unit Delay3/1
  icing/1 -> Unit Delay4/1
  2-D Lookup Table/1 -> Mux1/1  "C_L_delta_e"
  2-D Lookup Table8/1 -> Mux1/9  "C_n_delta_r"
  2-D Lookup Table1/1 -> Mux1/2  "C_D_delta_e"
  2-D Lookup Table2/1 -> Mux1/3  "C_m_delta_e"
  2-D Lookup Table3/1 -> Mux1/4  "C_Y_delta_a"
  2-D Lookup Table4/1 -> Mux1/5  "C_Y_delta_r"
  2-D Lookup Table5/1 -> Mux1/6  "C_l_delta_a"
  2-D Lookup Table6/1 -> Mux1/7  "C_l_delta_r"
  2-D Lookup Table7/1 -> Mux1/8  "C_n_delta_a"
  Unit Delay1/1 -> 2-D Lookup Table2/1, 2-D Lookup Table1/1, 2-D Lookup Table/1
  Unit Delay2/1 -> 2-D Lookup Table3/1, 2-D Lookup Table7/1, 2-D Lookup Table5/1
  Unit Delay3/1 -> 2-D Lookup Table8/1, 2-D Lookup Table6/1, 2-D Lookup Table4/1
  Unit Delay4/1 -> 2-D Lookup Table/2, 2-D Lookup Table1/2, 2-D Lookup Table2/2, 2-D Lookup Table3/2, 2-D Lookup Table5/2, 2-D Lookup Table6/2, 2-D Lookup Table7/2, 2-D Lookup Table8/2, 2-D Lookup Table4/2

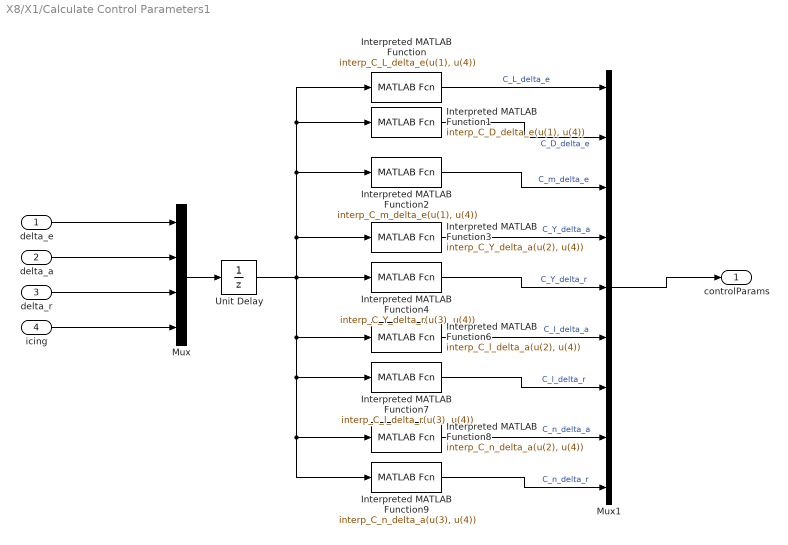
== system X8/X1/Calculate Control Parameters1 ==
  "delta_e " : Inport
  delta_a : Inport  Port=2
  "delta_r " : Inport  Port=3
  icing : Inport  Port=4
  Interpreted MATLAB Function : MATLABFcn  MATLABFcn=interp_C_L_delta_e(u(1), u(4))  OutputDimensions=1
  Interpreted MATLAB Function1 : MATLABFcn  MATLABFcn=interp_C_D_delta_e(u(1), u(4))  OutputDimensions=1
  Interpreted MATLAB Function2 : MATLABFcn  MATLABFcn=interp_C_m_delta_e(u(1), u(4))
  Interpreted MATLAB Function3 : MATLABFcn  MATLABFcn=interp_C_Y_delta_a(u(2), u(4))
  Interpreted MATLAB Function4 : MATLABFcn  MATLABFcn=interp_C_Y_delta_r(u(3), u(4))
  Interpreted MATLAB Function6 : MATLABFcn  MATLABFcn=interp_C_l_delta_a(u(2), u(4))
  Interpreted MATLAB Function7 : MATLABFcn  MATLABFcn=interp_C_l_delta_r(u(3), u(4))
  Interpreted MATLAB Function8 : MATLABFcn  MATLABFcn=interp_C_n_delta_a(u(2), u(4))
  Interpreted MATLAB Function9 : MATLABFcn  MATLABFcn=interp_C_n_delta_a(u(3), u(4))
  Mux : Mux
  Mux1 : Mux  Inputs=9
  Unit Delay : UnitDelay  SampleTime=-1  HasFrameUpgradeWarning=on
  controlParams : Outport  VectorParamsAs1DForOutWhenUnconnected=off
  wires:
  Mux/1 -> Unit Delay/1
  Mux1/1 -> controlParams/1
  Unit Delay/1 -> Interpreted MATLAB Function9/1, Interpreted MATLAB Function8/1, Interpreted MATLAB Function7/1, Interpreted MATLAB Function6/1, Interpreted MATLAB Function4/1, Interpreted MATLAB Function3/1, Interpreted MATLAB Function2/1, Interpreted MATLAB Function/1, Interpreted MATLAB Function1/1
  "delta_e "/1 -> Mux/1
  delta_a/1 -> Mux/2
  "delta_r "/1 -> Mux/3
  icing/1 -> Mux/4
  Interpreted MATLAB Function/1 -> Mux1/1  "C_L_delta_e"
  Interpreted MATLAB Function9/1 -> Mux1/9  "C_n_delta_r"
  Interpreted MATLAB Function1/1 -> Mux1/2  "C_D_delta_e"
  Interpreted MATLAB Function2/1 -> Mux1/3  "C_m_delta_e"
  Interpreted MATLAB Function3/1 -> Mux1/4  "C_Y_delta_a"
  Interpreted MATLAB Function4/1 -> Mux1/5  "C_Y_delta_r"
  Interpreted MATLAB Function6/1 -> Mux1/6  "C_l_delta_a"
  Interpreted MATLAB Function7/1 -> Mux1/7  "C_l_delta_r"
  Interpreted MATLAB Function8/1 -> Mux1/8  "C_n_delta_a"

== system X8/X1/Calculate Stability Parameters ==
  "alpha " : Inport
  beta : Inport  Port=2
  icing : Inport  Port=3
  Bus Creator : BusCreator  Inputs=2
  Interpreted MATLAB Function : MATLABFcn  Commented=on  MATLABFcn=interp_C_L_alpha(u(1), u(3))  OutputDimensions=1
  Interpreted MATLAB Function1 : MATLABFcn  Commented=on  MATLABFcn=interp_C_L_q(u(1), u(3))  OutputDimensions=1
  MATLAB Function1 : MATLAB Function  Commented=on  TreatAsAtomicUnit=on
  Saturation : Saturate  UpperLimit=deg2rad(15)  LowerLimit=deg2rad(-10)
  Saturation1 : Saturate  UpperLimit=deg2rad(15)  LowerLimit=deg2rad(-15)
  Subsystem : Subsystem
  Subsystem1 : Subsystem
  Unit Delay : UnitDelay  SampleTime=-1  HasFrameUpgradeWarning=on
  Unit Delay1 : UnitDelay  SampleTime=-1  HasFrameUpgradeWarning=on
  stabilityParams : Outport  VectorParamsAs1DForOutWhenUnconnected=off
  wires:
  "alpha "/1 -> Saturation/1
  beta/1 -> Saturation1/1
  Bus Creator/1 -> stabilityParams/1
  icing/1 -> Subsystem1/2(icing), Subsystem/2(icing)
  Subsystem1/1(Out1) -> Bus Creator/2
  Subsystem/1(Out1) -> Bus Creator/1
  Saturation1/1 -> Unit Delay1/1
  Saturation/1 -> Unit Delay/1
  Unit Delay/1 -> Subsystem/1(alpha)
  Unit Delay1/1 -> Subsystem1/1(beta)

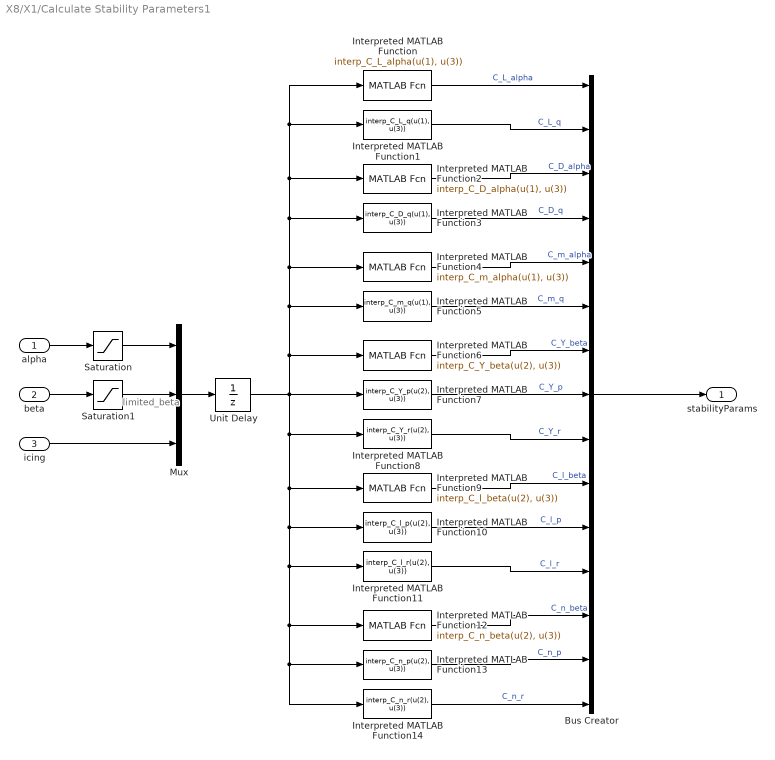
== system X8/X1/Calculate Stability Parameters1 ==
  note: limited_beta
  "alpha " : Inport
  beta : Inport  Port=2
  icing : Inport  Port=3
  Bus Creator : BusCreator  Inputs=15
  Interpreted MATLAB Function : MATLABFcn  MATLABFcn=interp_C_L_alpha(u(1), u(3))  OutputDimensions=1
  Interpreted MATLAB Function1 : MATLABFcn  MATLABFcn=interp_C_L_q(u(1), u(3))  OutputDimensions=1
  Interpreted MATLAB Function10 : MATLABFcn  MATLABFcn=interp_C_l_p(u(2), u(3))
  Interpreted MATLAB Function11 : MATLABFcn  MATLABFcn=interp_C_l_r(u(2), u(3))
  Interpreted MATLAB Function12 : MATLABFcn  MATLABFcn=interp_C_n_beta(u(2), u(3))
  Interpreted MATLAB Function13 : MATLABFcn  MATLABFcn=interp_C_n_p(u(2), u(3))
  Interpreted MATLAB Function14 : MATLABFcn  MATLABFcn=interp_C_n_r(u(2), u(3))
  Interpreted MATLAB Function2 : MATLABFcn  MATLABFcn=interp_C_D_alpha(u(1), u(3))
  Interpreted MATLAB Function3 : MATLABFcn  MATLABFcn=interp_C_D_q(u(1), u(3))
  Interpreted MATLAB Function4 : MATLABFcn  MATLABFcn=interp_C_m_alpha(u(1), u(3))
  Interpreted MATLAB Function5 : MATLABFcn  MATLABFcn=interp_C_m_q(u(1), u(3))
  Interpreted MATLAB Function6 : MATLABFcn  MATLABFcn=interp_C_Y_beta(u(2), u(3))
  Interpreted MATLAB Function7 : MATLABFcn  MATLABFcn=interp_C_Y_p(u(2), u(3))
  Interpreted MATLAB Function8 : MATLABFcn  MATLABFcn=interp_C_Y_r(u(2), u(3))
  Interpreted MATLAB Function9 : MATLABFcn  MATLABFcn=interp_C_l_beta(u(2), u(3))
  Mux : Mux  Inputs=3
  Saturation : Saturate  UpperLimit=deg2rad(15)  LowerLimit=deg2rad(-10)
  Saturation1 : Saturate  UpperLimit=deg2rad(15)  LowerLimit=deg2rad(-15)
  Unit Delay : UnitDelay  SampleTime=-1  HasFrameUpgradeWarning=on
  stabilityParams : Outport  VectorParamsAs1DForOutWhenUnconnected=off
  wires:
  "alpha "/1 -> Saturation/1
  beta/1 -> Saturation1/1
  icing/1 -> Mux/3
  Mux/1 -> Unit Delay/1
  Interpreted MATLAB Function/1 -> Bus Creator/1  "C_L_alpha"
  Interpreted MATLAB Function1/1 -> Bus Creator/2  "C_L_q"
  Interpreted MATLAB Function2/1 -> Bus Creator/3  "C_D_alpha"
  Interpreted MATLAB Function3/1 -> Bus Creator/4  "C_D_q"
  Interpreted MATLAB Function4/1 -> Bus Creator/5  "C_m_alpha"
  Interpreted MATLAB Function5/1 -> Bus Creator/6  "C_m_q"
  Bus Creator/1 -> stabilityParams/1
  Interpreted MATLAB Function6/1 -> Bus Creator/7  "C_Y_beta"
  Interpreted MATLAB Function8/1 -> Bus Creator/9  "C_Y_r"
  Interpreted MATLAB Function9/1 -> Bus Creator/10  "C_l_beta"
  Interpreted MATLAB Function7/1 -> Bus Creator/8  "C_Y_p"
  Interpreted MATLAB Function10/1 -> Bus Creator/11  "C_l_p"
  Interpreted MATLAB Function11/1 -> Bus Creator/12  "C_l_r"
  Interpreted MATLAB Function12/1 -> Bus Creator/13  "C_n_beta"
  Interpreted MATLAB Function13/1 -> Bus Creator/14  "C_n_p"
  Interpreted MATLAB Function14/1 -> Bus Creator/15  "C_n_r"
  Unit Delay/1 -> Interpreted MATLAB Function9/1, Interpreted MATLAB Function10/1, Interpreted MATLAB Function11/1, Interpreted MATLAB Function12/1, Interpreted MATLAB Function13/1, Interpreted MATLAB Function14/1, Interpreted MATLAB Function8/1, Interpreted MATLAB Function7/1, Interpreted MATLAB Function6/1, Interpreted MATLAB Function5/1, Interpreted MATLAB Function4/1, Interpreted MATLAB Function3/1, Interpreted MATLAB Function2/1, Interpreted MATLAB Function/1, Interpreted MATLAB Function1/1
  Saturation/1 -> Mux/1
  Saturation1/1 -> Mux/2
